simulink model "lab_5"  (R2015a)
settings: Solver=ode45  StartTime=0.0  StopTime=0.1  RelTol=1e-3
libraries: powerlib x8, powerlib_meascontrol x2
settings Model: Creator=DHARMIK  LastModifiedBy=DHARMIK

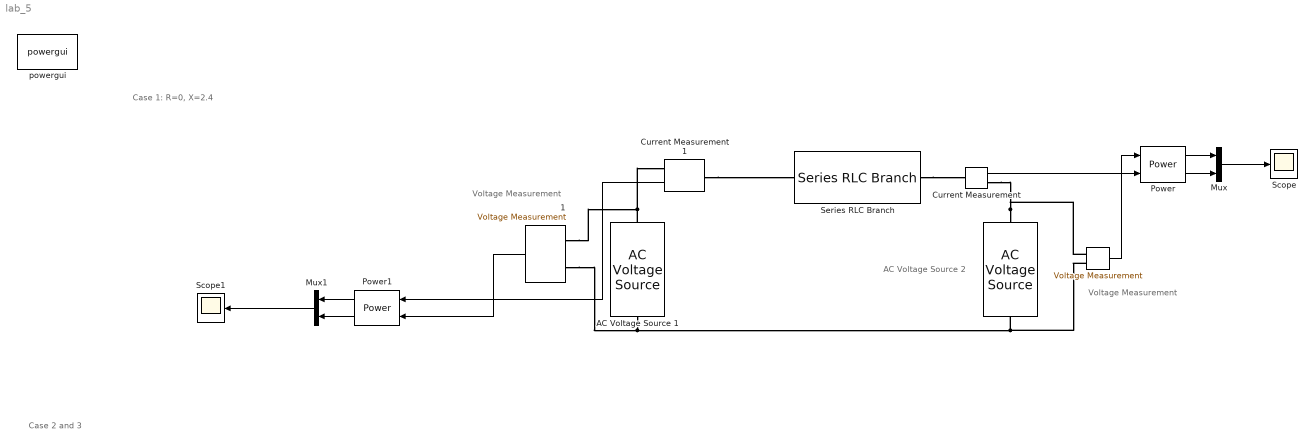
== system lab_5 ==
  note: Case 2 and 3
  note: Case 1: R=0, X=2.4
  note: Voltage Measurement
  note: AC Voltage Source 2
  note: Voltage Measurement
  " " : powerlib/Electrical Sources/AC Voltage Source  Amplitude=827.314  Phase=0  Frequency=50  SampleTime=0  Measurements=None
  " " : powerlib/Measurements/Voltage Measurement  PhasorSimulation=off  OutputType=Complex  PSBequivalent=0
  " 1" : powerlib/Measurements/Voltage Measurement  PhasorSimulation=off  OutputType=Complex  PSBequivalent=0
  AC Voltage Source 1 : powerlib/Electrical Sources/AC Voltage Source  Amplitude=707.106  Phase=16.26  Frequency=50  SampleTime=0  Measurements=None
  Current Measurement : powerlib/Measurements/Current Measurement  PhasorSimulation=off  OutputType=Complex  PSBequivalent=0
  Current Measurement1 : powerlib/Measurements/Current Measurement  PhasorSimulation=off  OutputType=Complex  PSBequivalent=0
  Mux : Mux  Inputs=2
  Mux1 : Mux  Inputs=2
  Power : powerlib_meascontrol/Measurements/Power  Freq=50  Vinit=[1, 0]  Iinit=[1, 0]  Ts=0
  Power1 : powerlib_meascontrol/Measurements/Power  Freq=50  Vinit=[1, 0]  Iinit=[1, 0]  Ts=0
  Scope : Scope
  Scope1 : Scope
      settings: YMin=0  YMax=0.5
  Series RLC Branch : powerlib/Elements/Series RLC Branch  LConnTagsString=__new0  RConnTagsString=__new0  BranchType=RL  Resistance=0  Inductance=0.0076394  SetiL0=off  InitialCurrent=0  Capacitance=0  Setx0=off  InitialVoltage=0  Measurements=None
  powergui : powerlib/powergui  Priority=1  SimulationMode=Discrete  SolverType=Tustin/Backward Euler (TBE)  SampleTime=50e-6  frequency=60  SPID=off  DisableSnubberDevices=off  DisableRonSwitches=off  DisableVfSwitches=off  SwTol=0  DisplayEquations=off  Interpol=off  methode=off  Ts=100  FunctionMessages=off  echomessages=off  HookPort=off  EnableUseOfTLC=off  x0status=blocks  frequencyindice=50  Pbase=100e6  ErrMax=1e-4  Iterations=50  UnitsV=kV  UnitsW=MW  buscounter=0  RestoreLinks=warning  ResistiveCurrentMeasurement=off  Frange=[0:2:500]  Ylog=off  Xlog=on  ShowGrid=off  save=off  variable=ZData  structure=0  ZoomFFT=off  StartTime=0.0  cycles=1  DisplayStyle=1  fundamental=60  FreqAxis=off  MaxFrequency=1000  frequencyindicesteady=1  RmsSteady=1  display=off
  wires:
  " "/1 -> Power/1
  Current Measurement/1 -> Power/2
  Power/1 -> Mux/1
  Power/2 -> Mux/2
  Mux/1 -> Scope/1
  " 1"/1 -> Power1/1
  Current Measurement1/1 -> Power1/2
  Power1/2 -> Mux1/1
  Power1/1 -> Mux1/2
  Mux1/1 -> Scope1/1
  connections:
  AC Voltage Source 1/RConn1 -- Current Measurement1/RConn1 -- " 1"/LConn2
  " "/RConn1 -- Current Measurement/RConn1 -- " "/LConn1
  AC Voltage Source 1/LConn1 -- " "/LConn2 -- " "/LConn1 -- " 1"/LConn1
  Series RLC Branch/RConn1 -- Current Measurement/LConn1
  Current Measurement1/LConn1 -- Series RLC Branch/LConn1
